simulink model "GCI_Ctrl_PLL_C2000"  (R2024a)
settings: Solver=FixedStepDiscrete  StartTime=0.0  StopTime=8  FixedStep=Sim.ContSampleTime  RelTol=1e-3  EnableMultiTasking=on
values from neighbouring files (symbols this model uses):
  ADPTV = 1.3912    [ModelDD.sldd]
  Ctrl = 0    [ModelDD.sldd]
  EnableMonitors = 0    [ModelDD.sldd]
  FrcPwr = 1    [ModelDD.sldd]
  IdSp = 0.0    [ModelDD.sldd]
  IqSp = 0.0    [ModelDD.sldd]
  ModReq = 1    [ModelDD.sldd]
  PorISel = 0    [ModelDD.sldd]
  PSp = 0.0    [ModelDD.sldd]
  QSp = 0.0    [ModelDD.sldd]
  Sim : value not decoded    [ModelDD.sldd]
  Test = 0    [ModelDD.sldd]
  Var = 650.0    [ModelDD.sldd]
undefined symbols (not defined in the file or in its folder): DiscIntNeverNeededParam, Down, GPTRIP1SEL, GPTRIP2SEL, magnitude, P, TZ1, TZ2, Up
libraries: simulink x38, c2837xDlib x22, c2802xlib x15, slpidlib x9, spsMeanLib x9, spsCurrentMeasurementLib x7, spsThreePhaseVIMeasurementLib x5, spsVoltageMeasurementLib x5, spsTHDLib x4, spsSeriesRLCBranchLib x4, svdutilitieslib x3, c280xlib x3
(part 6 of 11)

== system GCI_Ctrl_PLL_C2000/C2000_SW/CtrlLoop/ADC Scaling/ADC Scaling 3 Volts/Scaling2 ==
  CH : Inport
  Bias : Bias  Bias=-ADC_Off  SaturateOnIntegerOverflow=off
  Bias1 : Bias  Bias=-ADC_Off_Phy  SaturateOnIntegerOverflow=off
  Bus Creator : BusCreator  Inputs=2
  Data Type Conversion3 : DataTypeConversion  OutDataTypeStr=single  ConvertRealWorld=Stored Integer (SI)  SaturateOnIntegerOverflow=off  RndMeth=Floor
  Gain1 : Gain  Gain=ADC_Gain_Phy  OutDataTypeStr=single
  Gain2 : Gain  Gain=ADC_Gain  OutDataTypeStr=single
  Mon : Outport  VectorParamsAs1DForOutWhenUnconnected=off
  CH_Meas : Outport  Port=2  VectorParamsAs1DForOutWhenUnconnected=off
  wires:
  Gain1/1 -> Bus Creator/2, CH_Meas/1  "VcActMeas"
  Gain2/1 -> Bus Creator/1, Bias1/1  "VcPhyMeas"
  CH/1 -> Data Type Conversion3/1
  Data Type Conversion3/1 -> Bias/1
  Bias1/1 -> Gain1/1
  Bias/1 -> Gain2/1
  Bus Creator/1 -> Mon/1  "ScaleVcMon"

== system GCI_Ctrl_PLL_C2000/C2000_SW/CtrlLoop/ADC Scaling/ADC Scaling 3 Volts/Scaling3 ==
  CH : Inport
  Bias : Bias  Bias=-ADC_Off  SaturateOnIntegerOverflow=off
  Bias1 : Bias  Bias=-ADC_Off_Phy  SaturateOnIntegerOverflow=off
  Bus Creator : BusCreator  Inputs=2
  Data Type Conversion3 : DataTypeConversion  OutDataTypeStr=single  ConvertRealWorld=Stored Integer (SI)  SaturateOnIntegerOverflow=off  RndMeth=Floor
  Gain1 : Gain  Gain=ADC_Gain_Phy  OutDataTypeStr=single
  Gain2 : Gain  Gain=ADC_Gain  OutDataTypeStr=single
  Meas : Outport  VectorParamsAs1DForOutWhenUnconnected=off
  CH_Meas : Outport  Port=2  VectorParamsAs1DForOutWhenUnconnected=off
  wires:
  Gain1/1 -> Bus Creator/2, CH_Meas/1  "IaActMeas"
  Gain2/1 -> Bus Creator/1, Bias1/1  "IaPhyMeas"
  CH/1 -> Data Type Conversion3/1
  Data Type Conversion3/1 -> Bias/1
  Bias1/1 -> Gain1/1
  Bias/1 -> Gain2/1
  Bus Creator/1 -> Meas/1  "ScaleIaMon"

== system GCI_Ctrl_PLL_C2000/C2000_SW/CtrlLoop/ADC Scaling/ADC Scaling 3 Volts/Scaling4 ==
  CH : Inport
  Bias : Bias  Bias=-ADC_Off  SaturateOnIntegerOverflow=off
  Bias1 : Bias  Bias=-ADC_Off_Phy  SaturateOnIntegerOverflow=off
  Bus Creator : BusCreator  Inputs=2
  Data Type Conversion3 : DataTypeConversion  OutDataTypeStr=single  ConvertRealWorld=Stored Integer (SI)  SaturateOnIntegerOverflow=off  RndMeth=Floor
  Gain1 : Gain  Gain=ADC_Gain_Phy  OutDataTypeStr=single
  Gain2 : Gain  Gain=ADC_Gain  OutDataTypeStr=single
  Meas : Outport  VectorParamsAs1DForOutWhenUnconnected=off
  CH_Meas : Outport  Port=2  VectorParamsAs1DForOutWhenUnconnected=off
  wires:
  Gain1/1 -> Bus Creator/2, CH_Meas/1  "IbActMeas"
  Gain2/1 -> Bus Creator/1, Bias1/1  "IbPhyMeas"
  CH/1 -> Data Type Conversion3/1
  Data Type Conversion3/1 -> Bias/1
  Bias1/1 -> Gain1/1
  Bias/1 -> Gain2/1
  Bus Creator/1 -> Meas/1  "ScaleIbMon"

== system GCI_Ctrl_PLL_C2000/C2000_SW/CtrlLoop/ADC Scaling/ADC Scaling 3 Volts/Scaling5 ==
  CH : Inport
  Bias : Bias  Bias=-ADC_Off  SaturateOnIntegerOverflow=off
  Bias1 : Bias  Bias=-ADC_Off_Phy  SaturateOnIntegerOverflow=off
  Bus Creator : BusCreator  Inputs=2
  Data Type Conversion3 : DataTypeConversion  OutDataTypeStr=single  ConvertRealWorld=Stored Integer (SI)  SaturateOnIntegerOverflow=off  RndMeth=Floor
  Gain1 : Gain  Gain=ADC_Gain_Phy  OutDataTypeStr=single
  Gain2 : Gain  Gain=ADC_Gain  OutDataTypeStr=single
  Meas : Outport  VectorParamsAs1DForOutWhenUnconnected=off
  CH_Meas : Outport  Port=2  VectorParamsAs1DForOutWhenUnconnected=off
  wires:
  Gain1/1 -> Bus Creator/2, CH_Meas/1  "VdcActMeas"
  Gain2/1 -> Bus Creator/1, Bias1/1  "VdcPhyMeas"
  CH/1 -> Data Type Conversion3/1
  Data Type Conversion3/1 -> Bias/1
  Bias1/1 -> Gain1/1
  Bias/1 -> Gain2/1
  Bus Creator/1 -> Meas/1  "ScaleVdcMon"

== system GCI_Ctrl_PLL_C2000/C2000_SW/CtrlLoop/ADC Scaling/ADC Scaling 3 Volts/Subsystem ==
  IabcActMeas : Inport
  Enable : EnablePort
  LPF : Subsystem  mask{Ts=1/(Var.PWM_Freq), w=single(2*pi*5), K=single(1), y_0=0}
      mask prompts: Ts "Sample Time (s)"; w "CutOff Freq (-3db) (rad/s)"; K "Gain"; y_0 "Initial output"
  Saturation : Saturate  UpperLimit=5  LowerLimit=-5
  Offset : Outport
  wires:
  IabcActMeas/1 -> LPF/1(VabcGrid)
  LPF/1(y) -> Saturation/1
  Saturation/1 -> Offset/1

== system GCI_Ctrl_PLL_C2000/C2000_SW/CtrlLoop/ADCs/SIM/ADC_SIM ==
  CH : Inport
  Bias : Bias  Bias=ADC_Off  SaturateOnIntegerOverflow=off
  Bus Creator : BusCreator  Inputs=2
  Data Type Conversion : DataTypeConversion  OutDataTypeStr=uint16  SaturateOnIntegerOverflow=off  RndMeth=Floor
  Data Type Conversion4 : DataTypeConversion  SaturateOnIntegerOverflow=off  RndMeth=Floor
  Data Type Conversion8 : DataTypeConversion  SaturateOnIntegerOverflow=off  RndMeth=Floor
  Gain1 : Gain  Gain=1/ADC_Gain  OutDataTypeStr=single
  Round : Rounding  Operator=round
  Saturation : Saturate  UpperLimit=Res-1  LowerLimit=0
  Mon : Outport  VectorParamsAs1DForOutWhenUnconnected=off
  CH_Meas : Outport  Port=2  VectorParamsAs1DForOutWhenUnconnected=off
  wires:
  Round/1 -> Saturation/1
  CH/1 -> Data Type Conversion8/1, Gain1/1
  Gain1/1 -> Bias/1
  Saturation/1 -> Data Type Conversion/1
  Bias/1 -> Round/1
  Data Type Conversion/1 -> CH_Meas/1, Data Type Conversion4/1
  Data Type Conversion8/1 -> Bus Creator/1  "Phy"
  Data Type Conversion4/1 -> Bus Creator/2  "ADC"
  Bus Creator/1 -> Mon/1

== system GCI_Ctrl_PLL_C2000/C2000_SW/CtrlLoop/ADCs/SIM/ADC_SIM1 ==
  CH : Inport
  Bias : Bias  Bias=ADC_Off  SaturateOnIntegerOverflow=off
  Bus Creator : BusCreator  Inputs=2
  Data Type Conversion : DataTypeConversion  OutDataTypeStr=uint16  SaturateOnIntegerOverflow=off  RndMeth=Floor
  Data Type Conversion4 : DataTypeConversion  SaturateOnIntegerOverflow=off  RndMeth=Floor
  Data Type Conversion8 : DataTypeConversion  SaturateOnIntegerOverflow=off  RndMeth=Floor
  Gain1 : Gain  Gain=1/ADC_Gain  OutDataTypeStr=single
  Round : Rounding  Operator=round
  Saturation : Saturate  UpperLimit=Res-1  LowerLimit=0
  Mon : Outport  VectorParamsAs1DForOutWhenUnconnected=off
  CH_Meas : Outport  Port=2  VectorParamsAs1DForOutWhenUnconnected=off
  wires:
  Bus Creator/1 -> Mon/1
  Data Type Conversion4/1 -> Bus Creator/2  "ADC"
  Data Type Conversion8/1 -> Bus Creator/1  "Phy"
  Data Type Conversion/1 -> Data Type Conversion4/1, CH_Meas/1
  Bias/1 -> Round/1
  Saturation/1 -> Data Type Conversion/1
  Gain1/1 -> Bias/1
  CH/1 -> Data Type Conversion8/1, Gain1/1
  Round/1 -> Saturation/1

== system GCI_Ctrl_PLL_C2000/C2000_SW/CtrlLoop/ADCs/SIM/ADC_SIM2 ==
  CH : Inport
  Bias : Bias  Bias=ADC_Off  SaturateOnIntegerOverflow=off
  Bus Creator : BusCreator  Inputs=2
  Data Type Conversion : DataTypeConversion  OutDataTypeStr=uint16  SaturateOnIntegerOverflow=off  RndMeth=Floor
  Data Type Conversion4 : DataTypeConversion  SaturateOnIntegerOverflow=off  RndMeth=Floor
  Data Type Conversion8 : DataTypeConversion  SaturateOnIntegerOverflow=off  RndMeth=Floor
  Gain1 : Gain  Gain=1/ADC_Gain  OutDataTypeStr=single
  Round : Rounding  Operator=round
  Saturation : Saturate  UpperLimit=Res-1  LowerLimit=0
  Mon : Outport  VectorParamsAs1DForOutWhenUnconnected=off
  CH_Meas : Outport  Port=2  VectorParamsAs1DForOutWhenUnconnected=off
  wires:
  Round/1 -> Saturation/1
  CH/1 -> Gain1/1, Data Type Conversion8/1
  Gain1/1 -> Bias/1
  Saturation/1 -> Data Type Conversion/1
  Bias/1 -> Round/1
  Data Type Conversion/1 -> CH_Meas/1, Data Type Conversion4/1  "IaRawMeas"
  Data Type Conversion8/1 -> Bus Creator/1  "Phy"
  Data Type Conversion4/1 -> Bus Creator/2  "ADC"
  Bus Creator/1 -> Mon/1  "AdcIaMon"

== system GCI_Ctrl_PLL_C2000/C2000_SW/CtrlLoop/ADCs/SIM/ADC_SIM3 ==
  CH : Inport
  Bias : Bias  Bias=ADC_Off  SaturateOnIntegerOverflow=off
  Bus Creator : BusCreator  Inputs=2
  Data Type Conversion : DataTypeConversion  OutDataTypeStr=uint16  SaturateOnIntegerOverflow=off  RndMeth=Floor
  Data Type Conversion4 : DataTypeConversion  SaturateOnIntegerOverflow=off  RndMeth=Floor
  Data Type Conversion8 : DataTypeConversion  SaturateOnIntegerOverflow=off  RndMeth=Floor
  Gain1 : Gain  Gain=1/ADC_Gain  OutDataTypeStr=single
  Round : Rounding  Operator=round
  Saturation : Saturate  UpperLimit=Res-1  LowerLimit=0
  Mon : Outport  VectorParamsAs1DForOutWhenUnconnected=off
  CH_Meas : Outport  Port=2  VectorParamsAs1DForOutWhenUnconnected=off
  wires:
  Bus Creator/1 -> Mon/1  "AdcIbMon"
  Data Type Conversion4/1 -> Bus Creator/2  "ADC"
  Data Type Conversion8/1 -> Bus Creator/1  "Phy"
  Data Type Conversion/1 -> Data Type Conversion4/1, CH_Meas/1  "IbRawMeas"
  Bias/1 -> Round/1
  Saturation/1 -> Data Type Conversion/1
  Gain1/1 -> Bias/1
  CH/1 -> Data Type Conversion8/1, Gain1/1
  Round/1 -> Saturation/1

== system GCI_Ctrl_PLL_C2000/C2000_SW/CtrlLoop/ADCs/SIM/ADC_SIM4 ==
  CH : Inport
  Bias : Bias  Bias=ADC_Off  SaturateOnIntegerOverflow=off
  Bus Creator : BusCreator  Inputs=2
  Data Type Conversion : DataTypeConversion  OutDataTypeStr=uint16  SaturateOnIntegerOverflow=off  RndMeth=Floor
  Data Type Conversion4 : DataTypeConversion  SaturateOnIntegerOverflow=off  RndMeth=Floor
  Data Type Conversion8 : DataTypeConversion  SaturateOnIntegerOverflow=off  RndMeth=Floor
  Gain1 : Gain  Gain=1/ADC_Gain  OutDataTypeStr=single
  Round : Rounding  Operator=round
  Saturation : Saturate  UpperLimit=Res-1  LowerLimit=0
  Mon : Outport  VectorParamsAs1DForOutWhenUnconnected=off
  CH_Meas : Outport  Port=2  VectorParamsAs1DForOutWhenUnconnected=off
  wires:
  Round/1 -> Saturation/1
  CH/1 -> Gain1/1, Data Type Conversion8/1
  Gain1/1 -> Bias/1
  Saturation/1 -> Data Type Conversion/1
  Bias/1 -> Round/1
  Data Type Conversion/1 -> CH_Meas/1, Data Type Conversion4/1
  Data Type Conversion8/1 -> Bus Creator/1  "Phy"
  Data Type Conversion4/1 -> Bus Creator/2  "ADC"
  Bus Creator/1 -> Mon/1  "AdcVcMon"

== system GCI_Ctrl_PLL_C2000/C2000_SW/CtrlLoop/ADCs/SIM/ADC_SIM5 ==
  CH : Inport
  Bias : Bias  Bias=ADC_Off  SaturateOnIntegerOverflow=off
  Bus Creator : BusCreator  Inputs=2
  Data Type Conversion : DataTypeConversion  OutDataTypeStr=uint16  SaturateOnIntegerOverflow=off  RndMeth=Floor
  Data Type Conversion4 : DataTypeConversion  SaturateOnIntegerOverflow=off  RndMeth=Floor
  Data Type Conversion8 : DataTypeConversion  SaturateOnIntegerOverflow=off  RndMeth=Floor
  Gain1 : Gain  Gain=1/ADC_Gain  OutDataTypeStr=single
  Round : Rounding  Operator=round
  Saturation : Saturate  UpperLimit=Res-1  LowerLimit=0
  Mon : Outport  VectorParamsAs1DForOutWhenUnconnected=off
  CH_Meas : Outport  Port=2  VectorParamsAs1DForOutWhenUnconnected=off
  wires:
  Round/1 -> Saturation/1
  CH/1 -> Gain1/1, Data Type Conversion8/1
  Gain1/1 -> Bias/1
  Saturation/1 -> Data Type Conversion/1
  Bias/1 -> Round/1
  Data Type Conversion/1 -> CH_Meas/1, Data Type Conversion4/1  "VdcRawMeas"
  Data Type Conversion8/1 -> Bus Creator/1  "Phy"
  Data Type Conversion4/1 -> Bus Creator/2  "ADC"
  Bus Creator/1 -> Mon/1  "AdcVdcMon"

== system GCI_Ctrl_PLL_C2000/C2000_SW/CtrlLoop/CurrentController/CurrentController/Subsystem ==
  Vabc : Inport
  Iabc : Inport  Port=2
  wtNow : Inport  Port=3
  PowerCalculation : Subsystem
  Selector{3,5..7} (4 alike) : Selector  InputPortWidth=3  IndexOptions=Index vector (dialog)  Indices=[1 2]  OutputSizes=1
  abc_dqz : Subsystem  VariantControl=Var.Pll.SOGISel == 2
  dd_dqz1 : Subsystem  VariantControl=Var.Pll.SOGISel == 2
  dd_dqz2 : Subsystem  VariantControl=Var.Pll.SOGISel == 2
  P0 : Outport  VectorParamsAs1DForOutWhenUnconnected=off
  Q0 : Outport  Port=2  VectorParamsAs1DForOutWhenUnconnected=off
  VdqzP : Outport  Port=3  VectorParamsAs1DForOutWhenUnconnected=off
  VdqzN : Outport  Port=4  VectorParamsAs1DForOutWhenUnconnected=off
  IdqzP : Outport  Port=5  VectorParamsAs1DForOutWhenUnconnected=off
  IdqzN : Outport  Port=6  VectorParamsAs1DForOutWhenUnconnected=off
  Idqz : Outport  Port=7  VectorParamsAs1DForOutWhenUnconnected=off
  wires:
  dd_dqz1/2(dqzN) -> VdqzN/1, Selector5/1
  PowerCalculation/2(Q0) -> Q0/1  "Q0"
  Selector3/1 -> PowerCalculation/1(VdqP)  "VdqP"
  PowerCalculation/1(P0) -> P0/1  "P0"
  dd_dqz1/1(dqzP) -> VdqzP/1, Selector3/1
  Selector7/1 -> PowerCalculation/4(IdqzN)  "IdqN"
  Selector6/1 -> PowerCalculation/3(IdqzP)  "IdqP"
  dd_dqz2/1(dqzP) -> IdqzP/1, Selector6/1
  Selector5/1 -> PowerCalculation/2(VdqN)  "VdqN"
  dd_dqz2/2(dqzN) -> IdqzN/1, Selector7/1
  Iabc/1 -> abc_dqz/1(abc), dd_dqz2/1(abc)
  Vabc/1 -> dd_dqz1/1(abc)
  abc_dqz/1(dqz) -> Idqz/1
  wtNow/1 -> abc_dqz/2(wtNow), dd_dqz1/2(wtNow), dd_dqz2/2(wtNow)

== system GCI_Ctrl_PLL_C2000/C2000_SW/CtrlLoop/CurrentController/CurrentController/Subsystem1 ==
  u : Inport
  Enable : EnablePort
  Discrete PID Controller2 : slpidlib/PID Controller  Controller=PI  Form=Parallel  TimeDomain=Discrete-time  UseExternalTs=off  SampleTime=-1  IntegratorMethod=Forward Euler  FilterMethod=Forward Euler  ControllerParametersSource=internal  P=Var.Pwr_Kp  I=Var.Pwr_Ki  UseKiTs=off  D=0  UseExternalDerivativeSource=off  N=100  UseFilter=on  TunerSelectOption=Transfer Function Based (PID Tuner App)  InitialConditionSource=internal  InitialConditionForIntegrator=0  InitialConditionForFilter=0  DifferentiatorICPrevScaledInput=0  ExternalReset=none  TrackingMode=off  Kt=1  LimitOutput=on  SatLimitsSource=internal  UpperSaturationLimit=50  LowerSaturationLimit=-50  LinearizeAsGain=on  AntiWindupMode=clamping  Kb=1  LimitIntegrator=off  UpperIntegratorSaturationLimit=inf  LowerIntegratorSaturationLimit=-inf  POutMin=[]  POutMax=[]  IOutMin=[]  IOutMax=[]  DOutMin=[]  DOutMax=[]  NOutMin=[]  NOutMax=[]  SumOutMin=[]  SumOutMax=[]  SaturationOutMin=[]  SaturationOutMax=[]  PParamMin=[]  PParamMax=[]  IParamMin=[]  IParamMax=[]  DParamMin=[]  DParamMax=[]  NParamMin=[]  NParamMax=[]  KbParamMin=[]  KbParamMax=[]  KtParamMin=[]  KtParamMax=[]  KbOutMin=[]  KbOutMax=[]  KtOutMin=[]  KtOutMax=[]  IntegratorOutMin=[]  IntegratorOutMax=[]  FilterOutMin=[]  FilterOutMax=[]  SumI1OutMin=[]  SumI1OutMax=[]  SumI2OutMin=[]  SumI2OutMax=[]  SumI3OutMin=[]  SumI3OutMax=[]  SumI4OutMin=[]  SumI4OutMax=[]  SumDOutMin=[]  SumDOutMax=[]  DifferentiatorOutMin=[]  DifferentiatorOutMax=[]  FilterDiffOutCoefMin=[]  FilterDiffOutCoefMax=[]  ReciprocalOutMin=[]  ReciprocalOutMax=[]  SumDenOutMin=[]  SumDenOutMax=[]  SumNumOutMin=[]  SumNumOutMax=[]  DivideOutMin=[]  DivideOutMax=[]  UdiffTsProdOutMin=[]  UdiffTsProdOutMax=[]  NTsProdOutMin=[]  NTsProdOutMax=[]  UintegralTsProdOutMin=[]  UintegralTsProdOutMax=[]  UngainTsProdOutMin=[]  UngainTsProdOutMax=[]  ClampingZeroOutDataTypeStr=Inherit: Inherit via back propagation  ClampingZeroOutMin=[]  ClampingZeroOutMax=[]  FilterDenConstantOutDataTypeStr=Inherit: Inherit via back propagation  FilterDenConstantOutMin=[]  FilterDenConstantOutMax=[]  PCopyOutDataTypeStr=Inherit: Inherit via back propagation  PCopyOutMin=[]  PCopyOutMax=[]  NCopyOutDataTypeStr=Inherit: Inherit via back propagation  NCopyOutMin=[]  NCopyOutMax=[]  IntegratorContinuousStateAttributes=''  IntegratorStateMustResolveToSignalObject=off  IntegratorRTWStateStorageClass=Auto  FilterContinuousStateAttributes=''  FilterStateMustResolveToSignalObject=off  FilterRTWStateStorageClass=Auto  ParallelPVariant=InternalParameters  IdealPVariant=Disabled  IVariant=InternalParameters  DVariant=Disabled  IntegratorVariant=Discrete  SatVariant=Enabled  AWVariant=DiscClampingParallel  PCopyVariant=Disabled  TRVariant=Disabled  FdbkBlocksVariant=Forward  IdealPFdbkVariant=Disabled  SatFdbkVariant=Disabled  DerivativeFilterVariant=Disabled  NVariant=Disabled  NCopyVariant=Disabled_SignalSpec  FilterICVariant=Disabled  IntegratorICVariant=InternalICs  ExternalResetVariant=Disabled  TRSumVariant=Passthrough  SumFdbkVariant=Disabled  SumVariant=Sum_PI  TsampFilterVariant=InternalTs  TsampNgainVariant=Passthrough  TsampIntegralVariant=Disabled_SignalSpec  ExternalSaturationOutDataTypeStr=Inherit: Same as second input  DerivativeSourceVariant=Disabled
  y : Outport
  wires:
  u/1 -> Discrete PID Controller2/1
  Discrete PID Controller2/1 -> y/1  "PqCtrl"

== system GCI_Ctrl_PLL_C2000/C2000_SW/CtrlLoop/CurrentController/CurrentController/Subsystem2 ==
  In1 : Inport
  Discrete-Time Integrator : DiscreteIntegrator  SampleTime=-1  ICPrevOutput=DiscIntNeverNeededParam  ICPrevScaledInput=DiscIntNeverNeededParam
  Gain2 : Gain  Gain=1/(4*10/Var.PWM_Freq)
  Sum : Sum  Inputs=|+-
  Unit Delay : UnitDelay  SampleTime=-1  HasFrameUpgradeWarning=on
  Out1 : Outport
  wires:
  Gain2/1 -> Discrete-Time Integrator/1
  Sum/1 -> Gain2/1
  Discrete-Time Integrator/1 -> Unit Delay/1, Out1/1
  In1/1 -> Sum/1
  Unit Delay/1 -> Sum/2

== system GCI_Ctrl_PLL_C2000/C2000_SW/CtrlLoop/CurrentController/CurrentController/dqz2abc_1 ==
  dqz : Inport  OutDataTypeStr=single  PortDimensions=3
  wtNext : Inport  Port=2  OutDataTypeStr=single  PortDimensions=1
  Subsystem : Subsystem
  Subsystem1 : Subsystem
  abc : Outport  OutDataTypeStr=single  VectorParamsAs1DForOutWhenUnconnected=off
  wires:
  Subsystem/1(abc) -> abc/1
  Subsystem1/1(alpha_beta) -> Subsystem/1(al_be_0)
  dqz/1 -> Subsystem1/1(dqz)
  wtNext/1 -> Subsystem1/2(Ang)

== system GCI_Ctrl_PLL_C2000/C2000_SW/CtrlLoop/CurrentController/CurrentControllerAdptv/MESO ==
  "$y_{d,k+1}$" : Inport
  "$y_{k+1}$" : Inport  Port=2
  Enable : EnablePort  StatesWhenEnabling=reset
  CFDL : Subsystem
      settings: PortSchema="{\"entries\":[{\"content\":{\"sides\":[{\"content\":{},\"type\":\"ConnectorPlacement.EquallySpacedRectSide\",\"uuid\":\"4c1fb61f-a0f1-4f80-ab51-c2d0415b84a6\"},{\"content\":{\"connectorIds\":[\"Out1\"],\"side\":\"RIGHT\"},\"type\":\"ConnectorPlacement.EquallySpacedRectSide\",\"uuid\":\"9ff873c7-4b85-44b5-a865-19257b102083\"},{\"content\":{\"connectorIds\":[\"In1\"],\"side\":\"TOP\"},\"type\":\"ConnectorPlacement.EquallySpacedRectSide\",\"uuid\":\"4ecfe992-8541-4b45-a10f-40e2da0f3929\"},{\"content\":{\"connectorIds\":[\"In2\"],\"side\":\"BOTTOM\"},\"type\":\"ConnectorPlacement.EquallySpacedRectSide\",\"uuid\":\"cf2b25dc-6a11-497d-a08b-e8cfaefe89b4\"}]},\"type\":\"ConnectorPlacement.EquallySpacedConnector\",\"uuid\":\"e86a82e8-eb91-4ff3-be09-30688b92dc55\"}],\"packageUris\":[\"http://schema.mathworks.com/mf0/Connector/R2020b\"],\"version\":\"1.0\"}"
  Deso : Subsystem
      settings: PortSchema="{\"entries\":[{\"content\":{\"sides\":[{\"content\":{\"connectorIds\":[\"In1\"]},\"type\":\"ConnectorPlacement.EquallySpacedRectSide\",\"uuid\":\"29901263-609b-4396-8a94-0f8a9c24ad65\"},{\"content\":{\"connectorIds\":[\"Out1\"],\"side\":\"RIGHT\"},\"type\":\"ConnectorPlacement.EquallySpacedRectSide\",\"uuid\":\"cdbaa60c-7ed8-4615-a85a-44f6a1658969\"},{\"content\":{\"connectorIds\":[\"In2\",\"In3\"],\"side\":\"TOP\"},\"type\":\"ConnectorPlacement.EquallySpacedRectSide\",\"uuid\":\"dd234b30-071e-488e-8ced-1c6b8b59dcc9\"},{\"content\":{\"connectorIds\":[\"In4\"],\"side\":\"BOTTOM\"},\"type\":\"ConnectorPlacement.EquallySpacedRectSide\",\"uuid\":\"38d647c0-cdf9-46cf-9e52-179a2c4bbe41\"}]},\"type\":\"ConnectorPlacement.EquallySpacedConnector\",\"uuid\":\"808275f9-6432-411e-b696-a81ba7edf0b3\"}],\"packageUris\":[\"http://schema.mathworks.com/mf0/Connector/R2020b\"],\"version\":\"1.0\"}"
  Divide : Product  Inputs=**
  Lambda : Subsystem
  Mag : Subsystem  Commented=on
  Mag1 : Subsystem  Commented=on
  Mag2 : Subsystem
  Reciprocal : Product  Inputs=/
  Subsystem : Subsystem
  Sum1 : Sum  Inputs=|++
  Sum5 : Sum  Inputs=-+|
  Unit Delay1 : UnitDelay  SampleTime=-1  HasFrameUpgradeWarning=on
  Unit Delay2 : UnitDelay  SampleTime=-1  HasFrameUpgradeWarning=on
  $u_k$ : Outport
  wires:
  Subsystem/1($u_k$) -> $u_k$/1, Deso/2(u_k), Unit Delay1/1  "$u_k$"
  Mag2/1(Abs) -> Sum1/2  "$|| \\hat{\\Phi}_{e,k}  ||$"
  Unit Delay1/1 -> Subsystem/2("$u_{k-1}$"), Deso/3(u_k-1), CFDL/1(u_k-1)  "$u_{k-1}$"
  CFDL/1(Phi_k) -> Mag2/1(in), Deso/1(Phi_k)  "$\\hat{\\Phi}_{e,k}$"
  Deso/1(Lk_-ve) -> Divide/1  "$-\\hat{L}_k$"
  Sum1/1 -> Reciprocal/1
  "$y_{d,k+1}$"/1 -> Sum5/1  "$y_{d,k+1}$"
  Sum5/1 -> Unit Delay2/1  "$e_{k+1}$"
  Reciprocal/1 -> Divide/2  "$\\frac{1}{\\lambda_k + || \\hat{\\Phi}_{e,k}  ||}$"
  "$y_{k+1}$"/1 -> Sum5/2  "$y_{k+1}$"
  Unit Delay2/1 -> CFDL/2(e_k), Deso/4(e_k)  "$e_k$"
  Lambda/1($\lambda_k$) -> Sum1/1  "$\\lambda_k$"
  Divide/1 -> Subsystem/1($v_k$)  "$v_k$"

== system GCI_Ctrl_PLL_C2000/C2000_SW/CtrlLoop/CurrentController/CurrentControllerAdptv/Phase2Line ==
  In : Inport
  Line : Subsystem  VariantControl="Sim.ADC_UabcSensor == \"Three Currents\""
  Phase : Subsystem  VariantControl="Sim.ADC_UabcSensor == \"Three Volts\""
  Out : Outport

== system GCI_Ctrl_PLL_C2000/C2000_SW/CtrlLoop/CurrentController/CurrentControllerAdptv/Subsystem ==
  Vabc : Inport
  Iabc : Inport  Port=2
  wtNow : Inport  Port=3
  PowerCalculation : Subsystem
  Selector{3,5..7} (4 alike) : Selector  InputPortWidth=3  IndexOptions=Index vector (dialog)  Indices=[1 2]  OutputSizes=1
  abc_dqz : Subsystem  VariantControl=Var.Pll.SOGISel == 2
  dd_dqz1 : Subsystem  VariantControl=Var.Pll.SOGISel == 2
  dd_dqz2 : Subsystem  VariantControl=Var.Pll.SOGISel == 2
  P0 : Outport  VectorParamsAs1DForOutWhenUnconnected=off
  Q0 : Outport  Port=2  VectorParamsAs1DForOutWhenUnconnected=off
  VdqzP : Outport  Port=3  VectorParamsAs1DForOutWhenUnconnected=off
  VdqzN : Outport  Port=4  VectorParamsAs1DForOutWhenUnconnected=off
  IdqzP : Outport  Port=5  VectorParamsAs1DForOutWhenUnconnected=off
  IdqzN : Outport  Port=6  VectorParamsAs1DForOutWhenUnconnected=off
  Idqz : Outport  Port=7  VectorParamsAs1DForOutWhenUnconnected=off
  wires:
  wtNow/1 -> dd_dqz2/2(wtNow), dd_dqz1/2(wtNow), abc_dqz/2(wtNow)
  abc_dqz/1(dqz) -> Idqz/1
  Vabc/1 -> dd_dqz1/1(abc)
  Iabc/1 -> dd_dqz2/1(abc), abc_dqz/1(abc)
  dd_dqz2/2(dqzN) -> Selector7/1, IdqzN/1
  Selector5/1 -> PowerCalculation/2(VdqN)  "VdqN"
  dd_dqz2/1(dqzP) -> Selector6/1, IdqzP/1
  Selector6/1 -> PowerCalculation/3(IdqzP)  "IdqP"
  Selector7/1 -> PowerCalculation/4(IdqzN)  "IdqN"
  dd_dqz1/1(dqzP) -> Selector3/1, VdqzP/1
  PowerCalculation/1(P0) -> P0/1  "P0"
  Selector3/1 -> PowerCalculation/1(VdqP)  "VdqP"
  PowerCalculation/2(Q0) -> Q0/1  "Q0"
  dd_dqz1/2(dqzN) -> Selector5/1, VdqzN/1

== system GCI_Ctrl_PLL_C2000/C2000_SW/CtrlLoop/CurrentController/CurrentControllerAdptv/Subsystem2 ==
  In1 : Inport
  Discrete-Time Integrator : DiscreteIntegrator  SampleTime=-1  ICPrevOutput=DiscIntNeverNeededParam  ICPrevScaledInput=DiscIntNeverNeededParam
  Gain2 : Gain  Gain=1/(4*10/Var.PWM_Freq)
  Sum : Sum  Inputs=|+-
  Unit Delay : UnitDelay  SampleTime=-1  HasFrameUpgradeWarning=on
  Out1 : Outport
  wires:
  Unit Delay/1 -> Sum/2
  In1/1 -> Sum/1
  Discrete-Time Integrator/1 -> Out1/1, Unit Delay/1
  Sum/1 -> Gain2/1
  Gain2/1 -> Discrete-Time Integrator/1

== system GCI_Ctrl_PLL_C2000/C2000_SW/CtrlLoop/CurrentController/CurrentControllerAdptv/dqz2abc_1 ==
  dqz : Inport  OutDataTypeStr=single  PortDimensions=3
  wtNext : Inport  Port=2  OutDataTypeStr=single  PortDimensions=1
  Subsystem : Subsystem
  Subsystem1 : Subsystem
  abc : Outport  OutDataTypeStr=single  VectorParamsAs1DForOutWhenUnconnected=off
  wires:
  wtNext/1 -> Subsystem1/2(Ang)
  dqz/1 -> Subsystem1/1(dqz)
  Subsystem1/1(alpha_beta) -> Subsystem/1(al_be_0)
  Subsystem/1(abc) -> abc/1

== system GCI_Ctrl_PLL_C2000/C2000_SW/CtrlLoop/CurrentController/CurrentControllerAdptv/dqz2abc_2 ==
  dqz : Inport  OutDataTypeStr=single  PortDimensions=3
  wtNext : Inport  Port=2  OutDataTypeStr=single  PortDimensions=1
  Subsystem : Subsystem
  Subsystem1 : Subsystem
  abc : Outport  OutDataTypeStr=single  VectorParamsAs1DForOutWhenUnconnected=off
  wires:
  Subsystem/1(abc) -> abc/1  "abc"
  Subsystem1/1(alpha_beta) -> Subsystem/1(al_be_0)
  dqz/1 -> Subsystem1/1(dqz)
  wtNext/1 -> Subsystem1/2(Ang)

== system GCI_Ctrl_PLL_C2000/C2000_SW/CtrlLoop/CurrentController/CurrentControllerAdptv2/LPF ==
  u : Inport
  Alpha : Gain  Gain=(2-w*Ts)/(2+w*Ts)
  Beta : Gain  Gain=(w*Ts)/(2+w*Ts)
  Delay1 : Delay  DelayLength=1  InitialCondition=y_0
  Delay2 : Delay  DelayLength=1
  Sum1 : Sum  Inputs=++|
  Sum2 : Sum  Inputs=|++
  y : Outport  VectorParamsAs1DForOutWhenUnconnected=off
  wires:
  u/1 -> Sum1/1, Delay2/1
  Delay1/1 -> Alpha/1  "y(n-1)"
  Alpha/1 -> Sum2/2
  Delay2/1 -> Sum1/2
  Sum1/1 -> Beta/1
  Beta/1 -> Sum2/1
  Sum2/1 -> Delay1/1, y/1

== system GCI_Ctrl_PLL_C2000/C2000_SW/CtrlLoop/CurrentController/CurrentControllerAdptv2/MESO ==
  "$y_{d,k+1}$" : Inport
  "$y_{k+1}$" : Inport  Port=2
  CFDL : Subsystem
      settings: PortSchema="{\"entries\":[{\"content\":{\"sides\":[{\"content\":{},\"type\":\"ConnectorPlacement.EquallySpacedRectSide\",\"uuid\":\"4c1fb61f-a0f1-4f80-ab51-c2d0415b84a6\"},{\"content\":{\"connectorIds\":[\"Out1\"],\"side\":\"RIGHT\"},\"type\":\"ConnectorPlacement.EquallySpacedRectSide\",\"uuid\":\"9ff873c7-4b85-44b5-a865-19257b102083\"},{\"content\":{\"connectorIds\":[\"In1\"],\"side\":\"TOP\"},\"type\":\"ConnectorPlacement.EquallySpacedRectSide\",\"uuid\":\"4ecfe992-8541-4b45-a10f-40e2da0f3929\"},{\"content\":{\"connectorIds\":[\"In2\"],\"side\":\"BOTTOM\"},\"type\":\"ConnectorPlacement.EquallySpacedRectSide\",\"uuid\":\"cf2b25dc-6a11-497d-a08b-e8cfaefe89b4\"}]},\"type\":\"ConnectorPlacement.EquallySpacedConnector\",\"uuid\":\"e86a82e8-eb91-4ff3-be09-30688b92dc55\"}],\"packageUris\":[\"http://schema.mathworks.com/mf0/Connector/R2020b\"],\"version\":\"1.0\"}"
  Deso : Subsystem
      settings: PortSchema="{\"entries\":[{\"content\":{\"sides\":[{\"content\":{\"connectorIds\":[\"In1\"]},\"type\":\"ConnectorPlacement.EquallySpacedRectSide\",\"uuid\":\"29901263-609b-4396-8a94-0f8a9c24ad65\"},{\"content\":{\"connectorIds\":[\"Out1\"],\"side\":\"RIGHT\"},\"type\":\"ConnectorPlacement.EquallySpacedRectSide\",\"uuid\":\"cdbaa60c-7ed8-4615-a85a-44f6a1658969\"},{\"content\":{\"connectorIds\":[\"In2\",\"In3\"],\"side\":\"TOP\"},\"type\":\"ConnectorPlacement.EquallySpacedRectSide\",\"uuid\":\"dd234b30-071e-488e-8ced-1c6b8b59dcc9\"},{\"content\":{\"connectorIds\":[\"In4\"],\"side\":\"BOTTOM\"},\"type\":\"ConnectorPlacement.EquallySpacedRectSide\",\"uuid\":\"38d647c0-cdf9-46cf-9e52-179a2c4bbe41\"}]},\"type\":\"ConnectorPlacement.EquallySpacedConnector\",\"uuid\":\"808275f9-6432-411e-b696-a81ba7edf0b3\"}],\"packageUris\":[\"http://schema.mathworks.com/mf0/Connector/R2020b\"],\"version\":\"1.0\"}"
  Divide : Product  Inputs=**
  Lambda : Subsystem
  Mag : Subsystem  Commented=on
  Mag1 : Subsystem  Commented=on
  Mag2 : Subsystem
  Reciprocal : Product  Inputs=/
  Subsystem : Subsystem
  Sum1 : Sum  Inputs=|++
  Sum5 : Sum  Inputs=-+|
  Unit Delay1 : UnitDelay  SampleTime=-1  HasFrameUpgradeWarning=on
  Unit Delay2 : UnitDelay  SampleTime=-1  HasFrameUpgradeWarning=on
  $u_k$ : Outport
  wires:
  Divide/1 -> Subsystem/1($v_k$)  "$v_k$"
  Lambda/1($\lambda_k$) -> Sum1/1  "$\\lambda_k$"
  Unit Delay2/1 -> Deso/4(e_k), CFDL/2(e_k)  "$e_k$"
  "$y_{k+1}$"/1 -> Sum5/2  "$y_{k+1}$"
  Reciprocal/1 -> Divide/2  "$\\frac{1}{\\lambda_k + || \\hat{\\Phi}_{e,k}  ||}$"
  Sum5/1 -> Unit Delay2/1  "$e_{k+1}$"
  "$y_{d,k+1}$"/1 -> Sum5/1  "$y_{d,k+1}$"
  Sum1/1 -> Reciprocal/1
  Deso/1(Lk_-ve) -> Divide/1  "$-\\hat{L}_k$"
  CFDL/1(Phi_k) -> Deso/1(Phi_k), Mag2/1(in)  "$\\hat{\\Phi}_{e,k}$"
  Unit Delay1/1 -> CFDL/1(u_k-1), Deso/3(u_k-1), Subsystem/2("$u_{k-1}$")  "$u_{k-1}$"
  Mag2/1(Abs) -> Sum1/2  "$|| \\hat{\\Phi}_{e,k}  ||$"
  Subsystem/1($u_k$) -> Unit Delay1/1, Deso/2(u_k), $u_k$/1  "$u_k$"

== system GCI_Ctrl_PLL_C2000/C2000_SW/CtrlLoop/CurrentController/CurrentControllerAdptv2/Subsystem ==
  Vabc : Inport
  Iabc : Inport  Port=2
  wtNow : Inport  Port=3
  PowerCalculation : Subsystem
  Selector{3,5..7} (4 alike) : Selector  InputPortWidth=3  IndexOptions=Index vector (dialog)  Indices=[1 2]  OutputSizes=1
  abc_dqz : Subsystem  VariantControl=Var.Pll.SOGISel == 2
  abc_dqz1 : Subsystem  VariantControl=Var.Pll.SOGISel == 2
  dd_dqz1 : Subsystem  VariantControl=Var.Pll.SOGISel == 2
  dd_dqz2 : Subsystem  VariantControl=Var.Pll.SOGISel == 2
  P0 : Outport  VectorParamsAs1DForOutWhenUnconnected=off
  Q0 : Outport  Port=2  VectorParamsAs1DForOutWhenUnconnected=off
  VdqzP : Outport  Port=3  VectorParamsAs1DForOutWhenUnconnected=off
  VdqzN : Outport  Port=4  VectorParamsAs1DForOutWhenUnconnected=off
  IdqzP : Outport  Port=5  VectorParamsAs1DForOutWhenUnconnected=off
  IdqzN : Outport  Port=6  VectorParamsAs1DForOutWhenUnconnected=off
  Idqz : Outport  Port=7  VectorParamsAs1DForOutWhenUnconnected=off
  Vdqz : Outport  Port=8  VectorParamsAs1DForOutWhenUnconnected=off
  wires:
  dd_dqz1/2(dqzN) -> VdqzN/1, Selector5/1
  PowerCalculation/2(Q0) -> Q0/1  "Q0"
  Selector3/1 -> PowerCalculation/1(VdqP)  "VdqP"
  PowerCalculation/1(P0) -> P0/1  "P0"
  dd_dqz1/1(dqzP) -> VdqzP/1, Selector3/1
  Selector7/1 -> PowerCalculation/4(IdqzN)  "IdqN"
  Selector6/1 -> PowerCalculation/3(IdqzP)  "IdqP"
  dd_dqz2/1(dqzP) -> IdqzP/1, Selector6/1
  Selector5/1 -> PowerCalculation/2(VdqN)  "VdqN"
  dd_dqz2/2(dqzN) -> IdqzN/1, Selector7/1
  Iabc/1 -> abc_dqz/1(abc), dd_dqz2/1(abc)
  Vabc/1 -> abc_dqz1/1(abc), dd_dqz1/1(abc)
  wtNow/1 -> abc_dqz1/2(wtNow), abc_dqz/2(wtNow), dd_dqz1/2(wtNow), dd_dqz2/2(wtNow)
  abc_dqz/1(dqz) -> Idqz/1
  abc_dqz1/1(dqz) -> Vdqz/1

== system GCI_Ctrl_PLL_C2000/C2000_SW/CtrlLoop/CurrentController/CurrentControllerAdptv2/Subsystem1 ==
  PQ_sp : Inport
  Vdq : Inport  Port=2
  Divide1 : Product  Inputs=*/
  Gain1 : Gain  Gain=[1 -1]
  Gain2 : Gain  Gain=single(2/3)
  Matrix Concatenate : Concatenate  Mode=Multidimensional array  ConcatenateDimension=2
  Matrix Multiply : Product  Multiplication=Matrix(*)
  Saturation : Saturate  UpperLimit=inf  LowerLimit=1
  Selector1 : Selector  InputPortWidth=3  IndexOptions=Index vector (dialog)  Indices=[1 2]  OutputSizes=1
  Selector3 : Selector  InputPortWidth=3  IndexOptions=Index vector (dialog)  Indices=[1 2]  OutputSizes=1
  Selector4 : Selector  InputPortWidth=3  IndexOptions=Index vector (dialog)  Indices=[2 1]  OutputSizes=1
  Square : Math  Operator=square
  Sum of Elements : Sum  Inputs=+
  Idq* : Outport
  wires:
  Matrix Concatenate/1 -> Divide1/1
  Vdq/1 -> Selector3/1, Selector4/1, Selector1/1
  Gain1/1 -> Matrix Concatenate/2
  Selector4/1 -> Gain1/1
  Selector3/1 -> Square/1
  Selector1/1 -> Matrix Concatenate/1
  Sum of Elements/1 -> Saturation/1
  Square/1 -> Sum of Elements/1
  PQ_sp/1 -> Gain2/1
  Saturation/1 -> Divide1/2
  Divide1/1 -> Matrix Multiply/1
  Gain2/1 -> Matrix Multiply/2
  Matrix Multiply/1 -> Idq*/1

== system GCI_Ctrl_PLL_C2000/C2000_SW/CtrlLoop/CurrentController/CurrentControllerAdptv2/dqz2abc_1 ==
  dqz : Inport  OutDataTypeStr=single  PortDimensions=3
  wtNext : Inport  Port=2  OutDataTypeStr=single  PortDimensions=1
  Subsystem : Subsystem
  Subsystem1 : Subsystem
  abc : Outport  OutDataTypeStr=single  VectorParamsAs1DForOutWhenUnconnected=off
  wires:
  Subsystem/1(abc) -> abc/1
  Subsystem1/1(alpha_beta) -> Subsystem/1(al_be_0)
  dqz/1 -> Subsystem1/1(dqz)
  wtNext/1 -> Subsystem1/2(Ang)

== system GCI_Ctrl_PLL_C2000/C2000_SW/CtrlLoop/CurrentController/CurrentControllerPosNegSeq/Phase2Line ==
  In : Inport
  Line : Subsystem  VariantControl="Sim.ADC_UabcSensor == \"Three Currents\""
  Phase : Subsystem  VariantControl="Sim.ADC_UabcSensor == \"Three Volts\""
  Out : Outport

== system GCI_Ctrl_PLL_C2000/C2000_SW/CtrlLoop/CurrentController/CurrentControllerPosNegSeq/Subsystem ==
  Vabc : Inport
  Iabc : Inport  Port=2
  wtNow : Inport  Port=3
  PowerCalculation : Subsystem
  Selector{3,5..7} (4 alike) : Selector  InputPortWidth=3  IndexOptions=Index vector (dialog)  Indices=[1 2]  OutputSizes=1
  abc_dqz : Subsystem  VariantControl=Var.Pll.SOGISel == 2
  dd_dqz1 : Subsystem  VariantControl=Var.Pll.SOGISel == 2
  dd_dqz2 : Subsystem  VariantControl=Var.Pll.SOGISel == 2
  P0 : Outport  VectorParamsAs1DForOutWhenUnconnected=off
  Q0 : Outport  Port=2  VectorParamsAs1DForOutWhenUnconnected=off
  VdqzP : Outport  Port=3  VectorParamsAs1DForOutWhenUnconnected=off
  VdqzN : Outport  Port=4  VectorParamsAs1DForOutWhenUnconnected=off
  IdqzP : Outport  Port=5  VectorParamsAs1DForOutWhenUnconnected=off
  IdqzN : Outport  Port=6  VectorParamsAs1DForOutWhenUnconnected=off
  Idqz : Outport  Port=7  VectorParamsAs1DForOutWhenUnconnected=off
  wires:
  dd_dqz1/2(dqzN) -> VdqzN/1, Selector5/1
  PowerCalculation/2(Q0) -> Q0/1  "Q0"
  Selector3/1 -> PowerCalculation/1(VdqP)  "VdqP"
  PowerCalculation/1(P0) -> P0/1  "P0"
  dd_dqz1/1(dqzP) -> VdqzP/1, Selector3/1
  Selector7/1 -> PowerCalculation/4(IdqzN)  "IdqN"
  Selector6/1 -> PowerCalculation/3(IdqzP)  "IdqP"
  dd_dqz2/1(dqzP) -> IdqzP/1, Selector6/1
  Selector5/1 -> PowerCalculation/2(VdqN)  "VdqN"
  dd_dqz2/2(dqzN) -> IdqzN/1, Selector7/1
  Iabc/1 -> abc_dqz/1(abc), dd_dqz2/1(abc)
  Vabc/1 -> dd_dqz1/1(abc)
  abc_dqz/1(dqz) -> Idqz/1
  wtNow/1 -> abc_dqz/2(wtNow), dd_dqz1/2(wtNow), dd_dqz2/2(wtNow)

== system GCI_Ctrl_PLL_C2000/C2000_SW/CtrlLoop/CurrentController/CurrentControllerPosNegSeq/Subsystem1 ==
  u : Inport
  Enable : EnablePort
  Discrete PID Controller2 : slpidlib/PID Controller  Controller=PI  Form=Parallel  TimeDomain=Discrete-time  UseExternalTs=off  SampleTime=-1  IntegratorMethod=Forward Euler  FilterMethod=Forward Euler  ControllerParametersSource=internal  P=Var.Pwr_Kp  I=Var.Pwr_Ki  UseKiTs=off  D=0  UseExternalDerivativeSource=off  N=100  UseFilter=on  TunerSelectOption=Transfer Function Based (PID Tuner App)  InitialConditionSource=internal  InitialConditionForIntegrator=0  InitialConditionForFilter=0  DifferentiatorICPrevScaledInput=0  ExternalReset=none  TrackingMode=off  Kt=1  LimitOutput=on  SatLimitsSource=internal  UpperSaturationLimit=50  LowerSaturationLimit=-50  LinearizeAsGain=on  AntiWindupMode=clamping  Kb=1  LimitIntegrator=off  UpperIntegratorSaturationLimit=inf  LowerIntegratorSaturationLimit=-inf  POutMin=[]  POutMax=[]  IOutMin=[]  IOutMax=[]  DOutMin=[]  DOutMax=[]  NOutMin=[]  NOutMax=[]  SumOutMin=[]  SumOutMax=[]  SaturationOutMin=[]  SaturationOutMax=[]  PParamMin=[]  PParamMax=[]  IParamMin=[]  IParamMax=[]  DParamMin=[]  DParamMax=[]  NParamMin=[]  NParamMax=[]  KbParamMin=[]  KbParamMax=[]  KtParamMin=[]  KtParamMax=[]  KbOutMin=[]  KbOutMax=[]  KtOutMin=[]  KtOutMax=[]  IntegratorOutMin=[]  IntegratorOutMax=[]  FilterOutMin=[]  FilterOutMax=[]  SumI1OutMin=[]  SumI1OutMax=[]  SumI2OutMin=[]  SumI2OutMax=[]  SumI3OutMin=[]  SumI3OutMax=[]  SumI4OutMin=[]  SumI4OutMax=[]  SumDOutMin=[]  SumDOutMax=[]  DifferentiatorOutMin=[]  DifferentiatorOutMax=[]  FilterDiffOutCoefMin=[]  FilterDiffOutCoefMax=[]  ReciprocalOutMin=[]  ReciprocalOutMax=[]  SumDenOutMin=[]  SumDenOutMax=[]  SumNumOutMin=[]  SumNumOutMax=[]  DivideOutMin=[]  DivideOutMax=[]  UdiffTsProdOutMin=[]  UdiffTsProdOutMax=[]  NTsProdOutMin=[]  NTsProdOutMax=[]  UintegralTsProdOutMin=[]  UintegralTsProdOutMax=[]  UngainTsProdOutMin=[]  UngainTsProdOutMax=[]  ClampingZeroOutDataTypeStr=Inherit: Inherit via back propagation  ClampingZeroOutMin=[]  ClampingZeroOutMax=[]  FilterDenConstantOutDataTypeStr=Inherit: Inherit via back propagation  FilterDenConstantOutMin=[]  FilterDenConstantOutMax=[]  PCopyOutDataTypeStr=Inherit: Inherit via back propagation  PCopyOutMin=[]  PCopyOutMax=[]  NCopyOutDataTypeStr=Inherit: Inherit via back propagation  NCopyOutMin=[]  NCopyOutMax=[]  IntegratorContinuousStateAttributes=''  IntegratorStateMustResolveToSignalObject=off  IntegratorRTWStateStorageClass=Auto  FilterContinuousStateAttributes=''  FilterStateMustResolveToSignalObject=off  FilterRTWStateStorageClass=Auto  ParallelPVariant=InternalParameters  IdealPVariant=Disabled  IVariant=InternalParameters  DVariant=Disabled  IntegratorVariant=Discrete  SatVariant=Enabled  AWVariant=DiscClampingParallel  PCopyVariant=Disabled  TRVariant=Disabled  FdbkBlocksVariant=Forward  IdealPFdbkVariant=Disabled  SatFdbkVariant=Disabled  DerivativeFilterVariant=Disabled  NVariant=Disabled  NCopyVariant=Disabled_SignalSpec  FilterICVariant=Disabled  IntegratorICVariant=InternalICs  ExternalResetVariant=Disabled  TRSumVariant=Passthrough  SumFdbkVariant=Disabled  SumVariant=Sum_PI  TsampFilterVariant=InternalTs  TsampNgainVariant=Passthrough  TsampIntegralVariant=Disabled_SignalSpec  ExternalSaturationOutDataTypeStr=Inherit: Same as second input  DerivativeSourceVariant=Disabled
  y : Outport
  wires:
  u/1 -> Discrete PID Controller2/1
  Discrete PID Controller2/1 -> y/1  "PqCtrl"

== system GCI_Ctrl_PLL_C2000/C2000_SW/CtrlLoop/CurrentController/CurrentControllerPosNegSeq/Subsystem2 ==
  In1 : Inport
  Discrete-Time Integrator : DiscreteIntegrator  SampleTime=-1  ICPrevOutput=DiscIntNeverNeededParam  ICPrevScaledInput=DiscIntNeverNeededParam
  Gain2 : Gain  Gain=1/(4*10/Var.PWM_Freq)
  Sum : Sum  Inputs=|+-
  Unit Delay : UnitDelay  SampleTime=-1  HasFrameUpgradeWarning=on
  Out1 : Outport
  wires:
  Gain2/1 -> Discrete-Time Integrator/1
  Sum/1 -> Gain2/1
  Discrete-Time Integrator/1 -> Unit Delay/1, Out1/1
  In1/1 -> Sum/1
  Unit Delay/1 -> Sum/2

== system GCI_Ctrl_PLL_C2000/C2000_SW/CtrlLoop/CurrentController/CurrentControllerPosNegSeq/Subsystem4 ==
  PQ_sp : Inport
  Vdq : Inport  Port=2
  Divide1 : Product  Inputs=*/
  Gain1 : Gain  Gain=[1 -1]
  Gain2 : Gain  Gain=single(2/3)
  Matrix Concatenate : Concatenate  Mode=Multidimensional array  ConcatenateDimension=2
  Matrix Multiply : Product  Multiplication=Matrix(*)
  Saturation : Saturate  UpperLimit=inf  LowerLimit=1
  Selector1 : Selector  InputPortWidth=3  IndexOptions=Index vector (dialog)  Indices=[1 2]  OutputSizes=1
  Selector3 : Selector  InputPortWidth=3  IndexOptions=Index vector (dialog)  Indices=[1 2]  OutputSizes=1
  Selector4 : Selector  InputPortWidth=3  IndexOptions=Index vector (dialog)  Indices=[2 1]  OutputSizes=1
  Square : Math  Operator=square
  Sum of Elements : Sum  Inputs=+
  Idq* : Outport
  wires:
  Matrix Concatenate/1 -> Divide1/1
  Vdq/1 -> Selector3/1, Selector4/1, Selector1/1
  Gain1/1 -> Matrix Concatenate/2
  Selector4/1 -> Gain1/1
  Selector3/1 -> Square/1
  Selector1/1 -> Matrix Concatenate/1
  Sum of Elements/1 -> Saturation/1
  Square/1 -> Sum of Elements/1
  PQ_sp/1 -> Gain2/1
  Saturation/1 -> Divide1/2
  Divide1/1 -> Matrix Multiply/1
  Gain2/1 -> Matrix Multiply/2
  Matrix Multiply/1 -> Idq*/1

== system GCI_Ctrl_PLL_C2000/C2000_SW/CtrlLoop/CurrentController/CurrentControllerPosNegSeq/dqz2abc_1 ==
  dqz : Inport  OutDataTypeStr=single  PortDimensions=3
  wtNext : Inport  Port=2  OutDataTypeStr=single  PortDimensions=1
  Subsystem : Subsystem
  Subsystem1 : Subsystem
  abc : Outport  OutDataTypeStr=single  VectorParamsAs1DForOutWhenUnconnected=off
  wires:
  Subsystem/1(abc) -> abc/1
  Subsystem1/1(alpha_beta) -> Subsystem/1(al_be_0)
  dqz/1 -> Subsystem1/1(dqz)
  wtNext/1 -> Subsystem1/2(Ang)

== system GCI_Ctrl_PLL_C2000/C2000_SW/CtrlLoop/CurrentController/CurrentControllerPosNegSeq/dqz2abc_2 ==
  dqz : Inport  OutDataTypeStr=single  PortDimensions=3
  wtNext : Inport  Port=2  OutDataTypeStr=single  PortDimensions=1
  Subsystem : Subsystem
  Subsystem1 : Subsystem
  abc : Outport  OutDataTypeStr=single  VectorParamsAs1DForOutWhenUnconnected=off
  wires:
  wtNext/1 -> Subsystem1/2(Ang)
  dqz/1 -> Subsystem1/1(dqz)
  Subsystem1/1(alpha_beta) -> Subsystem/1(al_be_0)
  Subsystem/1(abc) -> abc/1  "abc"

== system GCI_Ctrl_PLL_C2000/C2000_SW/CtrlLoop/CurrentController/FeedForward/Subsystem ==
  Vabc : Inport
  Iabc : Inport  Port=2
  wtNow : Inport  Port=3
  LPF : Subsystem  mask{Ts=1/(Var.PWM_Freq), w=single(1000), K=single(1), y_0=0}
      mask prompts: Ts "Sample Time (s)"; w "CutOff Freq (-3db) (rad/s)"; K "Gain"; y_0 "Initial output"
  LPF1 : Subsystem  mask{Ts=1/(Var.PWM_Freq), w=single(1000), K=single(1), y_0=0}
      mask prompts: Ts "Sample Time (s)"; w "CutOff Freq (-3db) (rad/s)"; K "Gain"; y_0 "Initial output"
  PowerCalculation : Subsystem
  Selector{3,5..7} (4 alike) : Selector  InputPortWidth=3  IndexOptions=Index vector (dialog)  Indices=[1 2]  OutputSizes=1
  abc_dqz : Subsystem  VariantControl=Var.Pll.SOGISel == 2
  dd_dqz1 : Subsystem  VariantControl=Var.Pll.SOGISel == 2
  dd_dqz2 : Subsystem  VariantControl=Var.Pll.SOGISel == 2
  P0 : Outport  VectorParamsAs1DForOutWhenUnconnected=off
  Q0 : Outport  Port=2  VectorParamsAs1DForOutWhenUnconnected=off
  VdqzP : Outport  Port=3  VectorParamsAs1DForOutWhenUnconnected=off
  VdqzN : Outport  Port=4  VectorParamsAs1DForOutWhenUnconnected=off
  IdqzP : Outport  Port=5  VectorParamsAs1DForOutWhenUnconnected=off
  IdqzN : Outport  Port=6  VectorParamsAs1DForOutWhenUnconnected=off
  Idqz : Outport  Port=7  VectorParamsAs1DForOutWhenUnconnected=off
  wires:
  dd_dqz1/2(dqzN) -> VdqzN/1, Selector5/1
  PowerCalculation/2(Q0) -> LPF1/1(u)  "Q0"
  Selector3/1 -> PowerCalculation/1(VdqP)  "VdqP"
  PowerCalculation/1(P0) -> LPF/1(u)  "P0"
  dd_dqz1/1(dqzP) -> VdqzP/1, Selector3/1
  Selector7/1 -> PowerCalculation/4(IdqzN)  "IdqN"
  Selector6/1 -> PowerCalculation/3(IdqzP)  "IdqP"
  dd_dqz2/1(dqzP) -> IdqzP/1, Selector6/1
  Selector5/1 -> PowerCalculation/2(VdqN)  "VdqN"
  dd_dqz2/2(dqzN) -> IdqzN/1, Selector7/1
  LPF/1(y) -> P0/1  "P0"
  LPF1/1(y) -> Q0/1  "Q0"
  Iabc/1 -> abc_dqz/1(abc), dd_dqz2/1(abc)
  Vabc/1 -> dd_dqz1/1(abc)
  abc_dqz/1(dqz) -> Idqz/1
  wtNow/1 -> abc_dqz/2(wtNow), dd_dqz1/2(wtNow), dd_dqz2/2(wtNow)

== system GCI_Ctrl_PLL_C2000/C2000_SW/CtrlLoop/CurrentController/FeedForward/Subsystem1 ==
  u : Inport
  Enable : EnablePort
  Discrete PID Controller2 : slpidlib/PID Controller  Controller=PI  Form=Parallel  TimeDomain=Discrete-time  UseExternalTs=off  SampleTime=-1  IntegratorMethod=Forward Euler  FilterMethod=Forward Euler  ControllerParametersSource=internal  P=single(1/100)  I=single(0.1)  UseKiTs=off  D=0  UseExternalDerivativeSource=off  N=100  UseFilter=on  TunerSelectOption=Transfer Function Based (PID Tuner App)  InitialConditionSource=internal  InitialConditionForIntegrator=0  InitialConditionForFilter=0  DifferentiatorICPrevScaledInput=0  ExternalReset=none  TrackingMode=off  Kt=1  LimitOutput=on  SatLimitsSource=internal  UpperSaturationLimit=50  LowerSaturationLimit=-50  LinearizeAsGain=on  AntiWindupMode=clamping  Kb=1  LimitIntegrator=off  UpperIntegratorSaturationLimit=inf  LowerIntegratorSaturationLimit=-inf  POutMin=[]  POutMax=[]  IOutMin=[]  IOutMax=[]  DOutMin=[]  DOutMax=[]  NOutMin=[]  NOutMax=[]  SumOutMin=[]  SumOutMax=[]  SaturationOutMin=[]  SaturationOutMax=[]  PParamMin=[]  PParamMax=[]  IParamMin=[]  IParamMax=[]  DParamMin=[]  DParamMax=[]  NParamMin=[]  NParamMax=[]  KbParamMin=[]  KbParamMax=[]  KtParamMin=[]  KtParamMax=[]  KbOutMin=[]  KbOutMax=[]  KtOutMin=[]  KtOutMax=[]  IntegratorOutMin=[]  IntegratorOutMax=[]  FilterOutMin=[]  FilterOutMax=[]  SumI1OutMin=[]  SumI1OutMax=[]  SumI2OutMin=[]  SumI2OutMax=[]  SumI3OutMin=[]  SumI3OutMax=[]  SumI4OutMin=[]  SumI4OutMax=[]  SumDOutMin=[]  SumDOutMax=[]  DifferentiatorOutMin=[]  DifferentiatorOutMax=[]  FilterDiffOutCoefMin=[]  FilterDiffOutCoefMax=[]  ReciprocalOutMin=[]  ReciprocalOutMax=[]  SumDenOutMin=[]  SumDenOutMax=[]  SumNumOutMin=[]  SumNumOutMax=[]  DivideOutMin=[]  DivideOutMax=[]  UdiffTsProdOutMin=[]  UdiffTsProdOutMax=[]  NTsProdOutMin=[]  NTsProdOutMax=[]  UintegralTsProdOutMin=[]  UintegralTsProdOutMax=[]  UngainTsProdOutMin=[]  UngainTsProdOutMax=[]  ClampingZeroOutDataTypeStr=Inherit: Inherit via back propagation  ClampingZeroOutMin=[]  ClampingZeroOutMax=[]  FilterDenConstantOutDataTypeStr=Inherit: Inherit via back propagation  FilterDenConstantOutMin=[]  FilterDenConstantOutMax=[]  PCopyOutDataTypeStr=Inherit: Inherit via back propagation  PCopyOutMin=[]  PCopyOutMax=[]  NCopyOutDataTypeStr=Inherit: Inherit via back propagation  NCopyOutMin=[]  NCopyOutMax=[]  IntegratorContinuousStateAttributes=''  IntegratorStateMustResolveToSignalObject=off  IntegratorRTWStateStorageClass=Auto  FilterContinuousStateAttributes=''  FilterStateMustResolveToSignalObject=off  FilterRTWStateStorageClass=Auto  ParallelPVariant=InternalParameters  IdealPVariant=Disabled  IVariant=InternalParameters  DVariant=Disabled  IntegratorVariant=Discrete  SatVariant=Enabled  AWVariant=DiscClampingParallel  PCopyVariant=Disabled  TRVariant=Disabled  FdbkBlocksVariant=Forward  IdealPFdbkVariant=Disabled  SatFdbkVariant=Disabled  DerivativeFilterVariant=Disabled  NVariant=Disabled  NCopyVariant=Disabled_SignalSpec  FilterICVariant=Disabled  IntegratorICVariant=InternalICs  ExternalResetVariant=Disabled  TRSumVariant=Passthrough  SumFdbkVariant=Disabled  SumVariant=Sum_PI  TsampFilterVariant=InternalTs  TsampNgainVariant=Passthrough  TsampIntegralVariant=Disabled_SignalSpec  ExternalSaturationOutDataTypeStr=Inherit: Same as second input  DerivativeSourceVariant=Disabled
  y : Outport
  wires:
  u/1 -> Discrete PID Controller2/1
  Discrete PID Controller2/1 -> y/1  "PqCtrl"

== system GCI_Ctrl_PLL_C2000/C2000_SW/CtrlLoop/Modulation/SPWM/Subsystem ==
  abc : Inport  PortDimensions=3
  Gain1 : Gain  Gain=single(2/3)  ParamDataTypeStr=single  SaturateOnIntegerOverflow=on  OutDataTypeStr=Inherit: Same as input
  Gain3 : Gain  Gain="single([ 1   -1/2   -1/2; 0   sqrt(3)/2   -sqrt(3)/2; 1/2  1/2  1/2 ] )"  Multiplication=Matrix(K*u) (u vector)  ParamDataTypeStr=single  SaturateOnIntegerOverflow=on  OutDataTypeStr=Inherit: Same as input
  al_be_0 : Outport  VectorParamsAs1DForOutWhenUnconnected=off
  wires:
  abc/1 -> Gain3/1
  Gain3/1 -> Gain1/1
  Gain1/1 -> al_be_0/1  "VgAlphaBetaZero"

== system GCI_Ctrl_PLL_C2000/C2000_SW/CtrlLoop/PLL_Vref/SRF_PLL/LPF ==
  u : Inport
  Alpha : Gain  Gain=(2-w*Ts)/(2+w*Ts)
  Beta : Gain  Gain=(w*Ts)/(2+w*Ts)
  Delay1 : Delay  DelayLength=1  InitialCondition=y_0
  Delay2 : Delay  DelayLength=1
  Sum1 : Sum  Inputs=++|
  Sum2 : Sum  Inputs=|++
  y : Outport  VectorParamsAs1DForOutWhenUnconnected=off
  wires:
  u/1 -> Sum1/1, Delay2/1
  Delay1/1 -> Alpha/1  "y(n-1)"
  Alpha/1 -> Sum2/2
  Delay2/1 -> Sum1/2
  Sum1/1 -> Beta/1
  Beta/1 -> Sum2/1
  Sum2/1 -> Delay1/1, y/1  "w_Filt_30rad_s"

== system GCI_Ctrl_PLL_C2000/C2000_SW/CtrlLoop/PLL_Vref/SRF_PLL/LPF1 ==
  u : Inport
  Alpha : Gain  Gain=(2-w*Ts)/(2+w*Ts)
  Beta : Gain  Gain=(w*Ts)/(2+w*Ts)
  Delay1 : Delay  DelayLength=1  InitialCondition=y_0
  Delay2 : Delay  DelayLength=1
  Sum1 : Sum  Inputs=++|
  Sum2 : Sum  Inputs=|++
  y : Outport  VectorParamsAs1DForOutWhenUnconnected=off
  wires:
  Sum2/1 -> y/1, Delay1/1  "VgQ_PuAbsFilt"
  Beta/1 -> Sum2/1
  Sum1/1 -> Beta/1
  Delay2/1 -> Sum1/2
  Alpha/1 -> Sum2/2
  Delay1/1 -> Alpha/1  "y(n-1)"
  u/1 -> Delay2/1, Sum1/1

== system GCI_Ctrl_PLL_C2000/C2000_SW/CtrlLoop/PLL_Vref/SRF_PLL/LPF2 ==
  u : Inport
  Alpha : Gain  Gain=(2-w*Ts)/(2+w*Ts)
  Beta : Gain  Gain=(w*Ts)/(2+w*Ts)
  Delay1 : Delay  DelayLength=1  InitialCondition=y_0
  Delay2 : Delay  DelayLength=1
  Sum1 : Sum  Inputs=++|
  Sum2 : Sum  Inputs=|++
  y : Outport  VectorParamsAs1DForOutWhenUnconnected=off
  wires:
  u/1 -> Sum1/1, Delay2/1
  Delay1/1 -> Alpha/1  "y(n-1)"
  Alpha/1 -> Sum2/2
  Delay2/1 -> Sum1/2
  Sum1/1 -> Beta/1
  Beta/1 -> Sum2/1
  Sum2/1 -> Delay1/1, y/1  "VgQ_PuAbsFilt"

== system GCI_Ctrl_PLL_C2000/C2000_SW/CtrlLoop/PLL_Vref/SRF_PLL/WrapZeroToTwoPi ==
  Ang : Inport
  Constant2 : Constant  Value=single(2*pi)  OutDataTypeStr=single
  Mod1 : Math  Operator=mod  SignedPower=on  OutDataTypeStr=single
  wtWraped : Outport  VectorParamsAs1DForOutWhenUnconnected=off
  wires:
  Constant2/1 -> Mod1/2
  Mod1/1 -> wtWraped/1  "wtNext"
  Ang/1 -> Mod1/1

== system GCI_Ctrl_PLL_C2000/C2000_SW/CtrlLoop/PLL_Vref/SRF_PLL/WrapedDiscIntegrator ==
  w : Inport
  Compare To Constant : simulink/Logic and Bit Operations/Compare To Constant  relop=>=  const=single(2*pi)  OutDataTypeStr=boolean
  Discrete-Time Integrator1 : DiscreteIntegrator  IntegratorMethod=Integration: Trapezoidal  gainval=single(1)  ExternalReset=rising  InitialConditionSource=external  SampleTime=-1  OutDataTypeStr=single  ShowStatePort=on  ICPrevOutput=DiscIntNeverNeededParam  ICPrevScaledInput=DiscIntNeverNeededParam
  Gain2 : Gain  Gain=(1/Var.PWM_Freq)  ParamDataTypeStr=single
  Sum : Sum  Inputs=++|
  WrapZeroToTwoPi : Subsystem
  wt_now : Outport  VectorParamsAs1DForOutWhenUnconnected=off
  wires:
  Discrete-Time Integrator1/1 -> wt_now/1  "wt_now"
  Compare To Constant/1 -> Discrete-Time Integrator1/2
  Discrete-Time Integrator1/State -> Sum/1, Compare To Constant/1
  w/1 -> Gain2/1, Discrete-Time Integrator1/1
  Gain2/1 -> Sum/2
  WrapZeroToTwoPi/1(wtWraped) -> Discrete-Time Integrator1/3
  Sum/1 -> WrapZeroToTwoPi/1(Ang)  "Ang"
